simulink model "TP1_MCC"  (R2017b)
settings: Solver=ode15s  StartTime=0.0  StopTime=0.2  RelTol=1e-3
InitFcn:
  | TP1_MCC_cst
undefined symbols (not defined in the file or in its folder): b, J, K, L, R
settings Model: Creator=GEII Robot  LastModifiedBy=GEII Robot

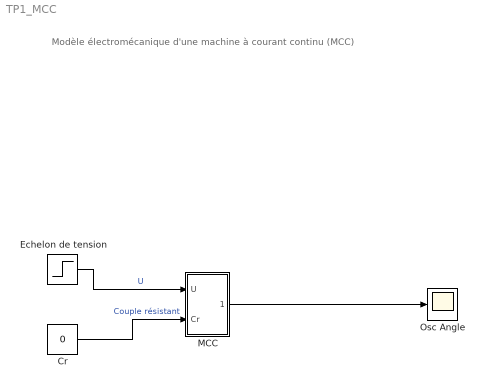
== system TP1_MCC ==
  note: Modèle électromécanique d'une machine à courant continu (MCC)
  Cr : Constant  Value=0
  Echelon de tension : Step  Time=0  After=12  SampleTime=0
  MCC : Subsystem
  Osc Angle : Scope
  wires:
  Echelon de tension/1 -> MCC/1(U)  "U"
  Cr/1 -> MCC/2(Cr)  "Couple résistant"
  MCC/1(theta) -> Osc Angle/1

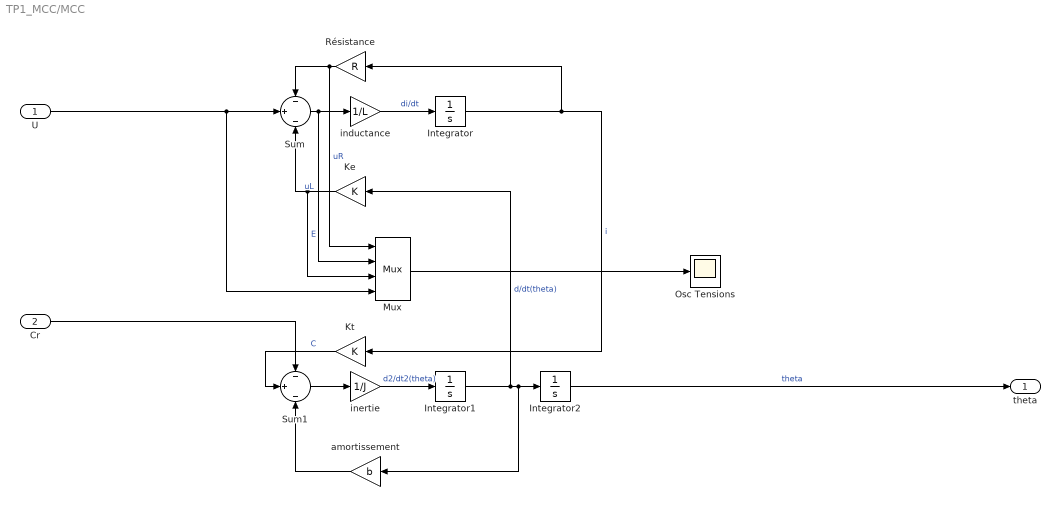
== system TP1_MCC/MCC ==
  U : Inport
  Cr : Inport  Port=2
  Integrator : Integrator
  Integrator1 : Integrator
  Integrator2 : Integrator
  Ke : Gain  Gain=K
  Kt : Gain  Gain=K
  Mux : Mux
      settings: DisplayOption=signals
  Osc Tensions : Scope
  Résistance : Gain  Gain=R
  Sum : Sum  Inputs=-|+|-
  Sum1 : Sum  Inputs=-|+|-
  amortissement : Gain  Gain=b
  inductance : Gain  Gain=1/L
  inertie : Gain  Gain=1/J
  theta : Outport
  wires:
  Cr/1 -> Sum1/1
  amortissement/1 -> Sum1/3
  Résistance/1 -> Mux/1, Sum/1  "uR"
  Integrator/1 -> Résistance/1, Kt/1  "i"
  Integrator2/1 -> theta/1  "theta"
  Ke/1 -> Mux/3, Sum/3  "E"
  U/1 -> Mux/4, Sum/2
  Integrator1/1 -> Ke/1, amortissement/1, Integrator2/1  "d/dt(theta)"
  Kt/1 -> Sum1/2  "C"
  Sum/1 -> Mux/2, inductance/1  "uL"
  inductance/1 -> Integrator/1  "di/dt"
  Mux/1 -> Osc Tensions/1
  inertie/1 -> Integrator1/1  "d2/dt2(theta)"
  Sum1/1 -> inertie/1
